simulink model "gm_sampleModel1786_sub"  (R2023a)
settings: Solver=VariableStepAuto  StartTime=0.0  StopTime=10.0  RelTol=1e-3
libraries: simulink x2
settings Model: Creator=user1  LastModifiedBy=user1
settings OptimizationCC: BlockReduction=off  ConditionallyExecuteInputs=off
settings DebuggingCC: InheritedTsInSrcMsg=none

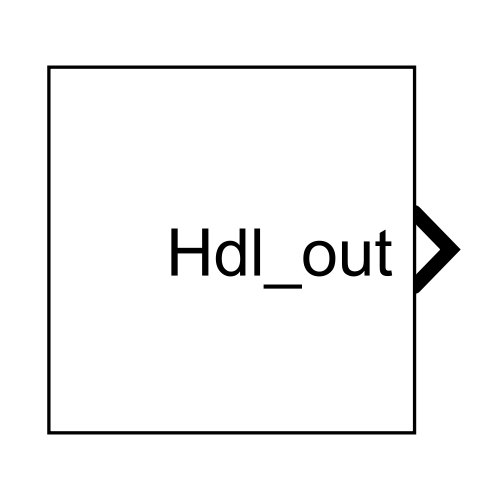
[thumbnail: Simulink's stored preview of the top-level diagram]
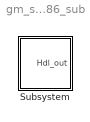
== system gm_sampleModel1786_sub ==
  Subsystem : Subsystem

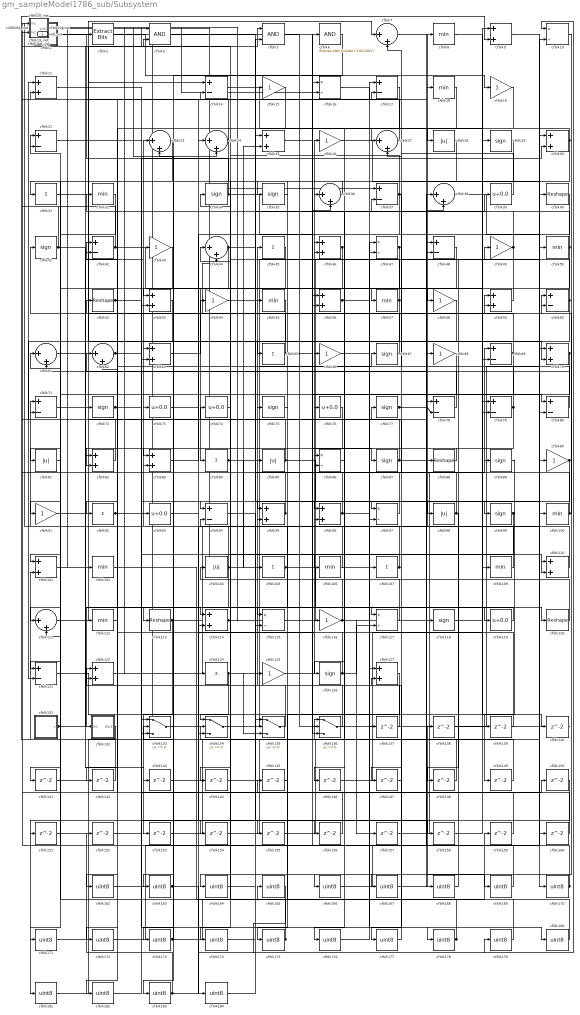
== system gm_sampleModel1786_sub/Subsystem ==
  cfblk1 : Subsystem  mask(Detect Rise Nonnegative){vinit=double(0), InputProcessing=Elements as channels (sample based), OutDataTypeStr=uint8}
      mask prompts: vinit "Simulink:masks:InitialCondition_MP"; InputProcessing "Simulink:masks:InputProcessing_MP"; OutDataTypeStr "Simulink:masks:OutputDataType_MP"
      mask help: Simulink:masks:DetectRiseNonnegative_MD
      mask init:
      | InputProcessing = 'Elements as channels (sample based)';
      | OutDataTypeStr = 'uint8';
      | vinit = double(0);
      mask TypeOptions InputProcessing: Simulink:masks:ColumnsAsChannelsFrameBased | Simulink:masks:ElementsAsChannelsSampleBased
      mask TypeOptions OutDataTypeStr: Simulink:masks:uint8 | Simulink:masks:boolean
      mask Display: fprintf('U >= 0\n&  NOT\nU/z >= 0')
  cfblk{10,16,47,86,97,115,117} (7 alike) : Product  Inputs=*/  OutDataTypeStr=uint8  RndMeth=Zero  SaturateOnIntegerOverflow=on
  cfblk{8,18,32,50,55,57,100,102,106,109,112} (11 alike) : MinMax  OutDataTypeStr=uint8
  cfblk{9,11,25,30,46,53,56,59,63,70,82..83,95..96,101,110,114,122,127} (19 alike) : Sum  OutDataTypeStr=uint8
  cfblk103_inst : Subsystem
  cfblk{28,81,85,98,104} (5 alike) : Abs  OutDataTypeStr=uint8  SaturateOnIntegerOverflow=off
  cfblk{31,45,65,84,92,105,107,124} (8 alike) : Sum  Inputs=+  OutDataTypeStr=uint8
  cfblk108_inst : Subsystem
  cfblk{7,23..24,27,36,38,44,61..62,111} (10 alike) : Sum  Inputs=|++  OutDataTypeStr=uint8
  cfblk{40,52,88,113,120} (5 alike) : Reshape
  cfblk{15,19,26,43,49,54,58,66,68,90..91,116,125} (13 alike) : Gain  OutDataTypeStr=uint8
  cfblk{29,34..35,41,67,72,75,77,87,89,99,118,126} (13 alike) : Signum
  cfblk{39,73..74,76,93,119} (6 alike) : Bias  Bias=0.0  SaturateOnIntegerOverflow=off
  cfblk{14,17,21,37,42,48,60,69,71,78..80,94,121} (14 alike) : Sum  Inputs=+-  OutDataTypeStr=uint8
  cfblk131 : Subsystem  mask(Counter Free-Running){NumBits=double(16), tsamp=double(-1)}
      mask prompts: NumBits "Simulink:masks:NumberOfBits_MP"; tsamp "Simulink:masks:SampleTime_MP"
      mask help: Simulink:masks:CounterFreeRunning_MD
  cfblk132 : Subsystem
  cfblk{133..136} (4 alike) : Switch  OutDataTypeStr=uint8  SaturateOnIntegerOverflow=off  InputSameDT=off
  cfblk{137..160} (24 alike) : Delay  SampleTime=1
  cfblk13_inst : Subsystem
  cfblk{162..184} (23 alike) : DataTypeConversion  OutDataTypeStr=uint8  SaturateOnIntegerOverflow=off  RndMeth=Floor
  cfblk2 : simulink/Logic and Bit Operations/Extract Bits  bitsToExtract=Upper half  numBits=8  bitIdxRange=[0 7]  outScalingMode=Preserve fixed-point scaling
      settings: LibrarySourceBlock=|
      | hdlsllib/Logic and Bit
      | Operations/Extract Bits
  cfblk20_inst : Subsystem
  cfblk22_inst : Subsystem
  cfblk3 : Logic  AllPortsSameDT=off  OutDataTypeStr=boolean
  cfblk4 : Constant  Value=0  OutDataTypeStr=uint8  SampleTime=1
  cfblk5 : Logic  AllPortsSameDT=off  OutDataTypeStr=boolean
  cfblk6 : simulink/Logic and Bit Operations/Bitwise Operator  logicop=AND  UseBitMask=on  BitMask=bin2dec('11011001')  BitMaskRealWorld=Stored Integer
      settings: LibrarySourceBlock=|
      | hdlsllib/Logic and Bit
      | Operations/Bitwise
      | Operator
  cfblk64_inst : Subsystem
  Hdl_out : Outport  OutDataTypeStr=uint8  SampleTime=1
  wires:
  cfblk1/1(Y) -> cfblk70/2, cfblk7/1, Hdl_out/1
  cfblk10/1 -> cfblk164/1
  cfblk100/1 -> cfblk60/1, cfblk108_inst/1(in1)
  cfblk101/1 -> cfblk5/1
  cfblk102/1 -> cfblk165/1
  cfblk103_inst/1(out1) -> cfblk72/1
  cfblk104/1 -> cfblk64_inst/2(in2), cfblk25/2, cfblk132/1(In1)
  cfblk105/1 -> cfblk67/1, cfblk120/1
  cfblk106/1 -> cfblk94/2
  cfblk107/1 -> cfblk23/1, cfblk26/1
  cfblk108_inst/1(out1) -> cfblk37/1, cfblk24/2, cfblk103_inst/2(in2)
  cfblk109/1 -> cfblk71/1
  cfblk11/1 -> cfblk53/2
  cfblk110/1 -> cfblk8/1
  cfblk111/1 -> cfblk78/1
  cfblk112/1 -> cfblk62/2
  cfblk113/1 -> cfblk153/1, cfblk117/1
  cfblk114/1 -> cfblk88/1, cfblk59/1
  cfblk115/1 -> cfblk49/1
  cfblk116/1 -> cfblk34/1, cfblk157/1
  cfblk117/1 -> cfblk76/1
  cfblk118/1 -> cfblk29/1
  cfblk119/1 -> cfblk113/1
  cfblk120/1 -> cfblk45/1
  cfblk121/1 -> cfblk149/1
  cfblk122/1 -> cfblk50/1
  cfblk124/1 -> cfblk60/2, cfblk40/1, cfblk135/3, cfblk134/1
  cfblk125/1 -> cfblk86/1
  cfblk126/1 -> cfblk52/1, cfblk117/2
  cfblk127/1 -> cfblk175/1
  cfblk13_inst/1(out1) -> cfblk16/2
  cfblk131/1(y) -> cfblk17/2, cfblk68/1
  cfblk132/1(Out1) -> cfblk9/2
  cfblk133/1 -> cfblk73/1
  cfblk134/1 -> cfblk66/1
  cfblk135/1 -> cfblk75/1
  cfblk136/1 -> cfblk42/1
  cfblk137/1 -> cfblk122/1
  cfblk138/1 -> cfblk70/1
  cfblk139/1 -> cfblk44/1
  cfblk14/1 -> cfblk109/1
  cfblk140/1 -> cfblk1/1(U)
  cfblk141/1 -> cfblk5/2
  cfblk142/1 -> cfblk101/2
  cfblk143/1 -> cfblk136/1
  cfblk144/1 -> cfblk97/2
  cfblk145/1 -> cfblk95/2
  cfblk146/1 -> cfblk9/1
  cfblk147/1 -> cfblk177/1
  cfblk148/1 -> cfblk134/2
  cfblk149/1 -> cfblk46/1
  cfblk15/1 -> cfblk183/1
  cfblk150/1 -> cfblk181/1
  cfblk151/1 -> cfblk47/2
  cfblk152/1 -> cfblk30/2
  cfblk153/1 -> cfblk136/2
  cfblk154/1 -> cfblk36/2
  cfblk155/1 -> cfblk80/2
  cfblk156/1 -> cfblk20_inst/2(in2)
  cfblk157/1 -> cfblk69/1
  cfblk158/1 -> cfblk79/1
  cfblk159/1 -> cfblk61/1
  cfblk16/1 -> cfblk137/1
  cfblk160/1 -> cfblk42/2
  cfblk162/1 -> cfblk6/1
  cfblk163/1 -> cfblk184/1, cfblk116/1
  cfblk164/1 -> cfblk89/1
  cfblk165/1 -> cfblk10/1
  cfblk166/1 -> cfblk10/2
  cfblk167/1 -> cfblk138/1
  cfblk168/1 -> cfblk48/1
  cfblk169/1 -> cfblk48/2
  cfblk17/1 -> cfblk112/1
  cfblk170/1 -> cfblk83/2, cfblk64_inst/1(in1)
  cfblk171/1 -> cfblk38/1
  cfblk172/1 -> cfblk38/2
  cfblk173/1 -> cfblk135/1, cfblk133/2, cfblk159/1
  cfblk174/1 -> cfblk55/1
  cfblk175/1 -> cfblk63/1, cfblk104/1
  cfblk176/1 -> cfblk127/1
  cfblk177/1 -> cfblk127/2
  cfblk178/1 -> cfblk71/2, cfblk145/1, cfblk125/1
  cfblk179/1 -> cfblk21/1
  cfblk18/1 -> cfblk63/2
  cfblk180/1 -> cfblk21/2
  cfblk181/1 -> cfblk115/2
  cfblk182/1 -> cfblk150/1
  cfblk183/1 -> cfblk96/2, cfblk179/1, cfblk152/1
  cfblk184/1 -> cfblk15/1
  cfblk19/1 -> cfblk126/1
  cfblk2/1 -> cfblk19/1
  cfblk20_inst/1(out1) -> cfblk135/2, cfblk107/1
  cfblk21/1 -> cfblk178/1
  cfblk22_inst/1(out1) -> cfblk102/1
  cfblk23/1 -> cfblk31/1
  cfblk24/1 -> cfblk82/2, cfblk22_inst/2(in2)
  cfblk25/1 -> cfblk28/1
  cfblk26/1 -> cfblk100/1
  cfblk27/1 -> cfblk16/1
  cfblk28/1 -> cfblk121/1
  cfblk29/1 -> cfblk65/1
  cfblk3/1 -> cfblk96/1
  cfblk30/1 -> cfblk27/1, cfblk162/1, cfblk144/1
  cfblk31/1 -> cfblk14/1
  cfblk32/1 -> cfblk151/1
  cfblk34/1 -> cfblk56/1, cfblk2/1
  cfblk35/1 -> cfblk95/1
  cfblk36/1 -> cfblk35/1
  cfblk37/1 -> cfblk3/2, cfblk134/3, cfblk97/1
  cfblk38/1 -> cfblk170/1
  cfblk39/1 -> cfblk14/2
  cfblk4/1 -> cfblk118/1
  cfblk40/1 -> cfblk166/1
  cfblk41/1 -> cfblk3/1, cfblk114/1, cfblk108_inst/2(in2)
  cfblk42/1 -> cfblk69/2, cfblk22_inst/1(in1), cfblk168/1
  cfblk43/1 -> cfblk111/2
  cfblk44/1 -> cfblk122/2, cfblk18/1
  cfblk45/1 -> cfblk53/1
  cfblk46/1 -> cfblk171/1, cfblk101/1
  cfblk47/1 -> cfblk46/2, cfblk172/1, cfblk84/1
  cfblk48/1 -> cfblk167/1
  cfblk49/1 -> cfblk182/1, cfblk32/1
  cfblk5/1 -> cfblk79/2
  cfblk50/1 -> cfblk37/2, cfblk57/1
  cfblk52/1 -> cfblk93/1, cfblk106/1
  cfblk53/1 -> cfblk141/1
  cfblk54/1 -> cfblk39/1
  cfblk55/1 -> cfblk173/1
  cfblk56/1 -> cfblk99/1, cfblk110/2
  cfblk57/1 -> cfblk136/3, cfblk13_inst/1(in1)
  cfblk58/1 -> cfblk92/1
  cfblk59/1 -> cfblk58/1
  cfblk6/1 -> cfblk163/1
  cfblk60/1 -> cfblk27/2, cfblk121/2
  cfblk61/1 -> cfblk44/2
  cfblk62/1 -> cfblk133/1, cfblk110/1
  cfblk63/1 -> cfblk54/1
  cfblk64_inst/1(out1) -> cfblk124/1
  cfblk65/1 -> cfblk87/1, cfblk25/1
  cfblk66/1 -> cfblk98/1
  cfblk67/1 -> cfblk41/1
  cfblk68/1 -> cfblk94/1
  cfblk69/1 -> cfblk81/1, cfblk91/1, cfblk47/1
  cfblk7/1 -> cfblk80/1
  cfblk70/1 -> cfblk61/2, cfblk114/2
  cfblk71/1 -> cfblk143/1
  cfblk72/1 -> cfblk59/2, cfblk30/1
  cfblk73/1 -> cfblk24/1
  cfblk74/1 -> cfblk174/1
  cfblk75/1 -> cfblk115/1
  cfblk76/1 -> cfblk83/1
  cfblk77/1 -> cfblk78/2, cfblk147/1
  cfblk78/1 -> cfblk62/1
  cfblk79/1 -> cfblk7/2, cfblk11/2, cfblk142/1
  cfblk8/1 -> cfblk140/1
  cfblk80/1 -> cfblk36/1
  cfblk81/1 -> cfblk111/1
  cfblk82/1 -> cfblk13_inst/2(in2)
  cfblk83/1 -> cfblk17/1
  cfblk84/1 -> cfblk56/2, cfblk105/1
  cfblk85/1 -> cfblk20_inst/1(in1), cfblk160/1
  cfblk86/1 -> cfblk176/1
  cfblk87/1 -> cfblk169/1, cfblk11/1
  cfblk88/1 -> cfblk82/1
  cfblk89/1 -> cfblk139/1
  cfblk9/1 -> cfblk90/1
  cfblk90/1 -> cfblk133/3, cfblk146/1
  cfblk91/1 -> cfblk43/1
  cfblk92/1 -> cfblk74/1, cfblk158/1
  cfblk93/1 -> cfblk155/1
  cfblk94/1 -> cfblk156/1
  cfblk95/1 -> cfblk85/1, cfblk23/2
  cfblk96/1 -> cfblk180/1, cfblk86/2
  cfblk97/1 -> cfblk103_inst/1(in1)
  cfblk98/1 -> cfblk77/1, cfblk148/1
  cfblk99/1 -> cfblk119/1, cfblk154/1

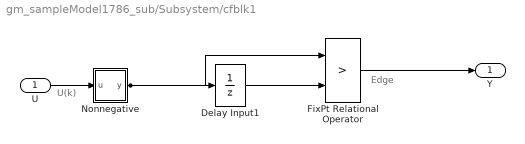
== system gm_sampleModel1786_sub/Subsystem/cfblk1 ==
  note: U(k)
  note: Edge
  U : Inport  OutDataTypeStr=uint8  SampleTime=1
  Delay Input1 : UnitDelay  Description=Store in Global RAM  DisableCoverage=on  InitialCondition=vinit  SampleTime=-1  HasFrameUpgradeWarning=on
  FixPt Relational Operator : RelationalOperator  Operator=>  OutDataTypeStr=fixdt(0, 8)  ZeroCross=off  InputSameDT=off
  Nonnegative : Subsystem  mask(Compare To Zero){relop=>=, OutDataTypeStr=boolean, ZeroCross=off}
      mask prompts: relop "Simulink:masks:Operator_MP"; OutDataTypeStr "Simulink:masks:OutputDataType_MP"; ZeroCross "Simulink:masks:EnableZerocrossingDetection_MP"
      mask help: Simulink:masks:CompareToZero_MD
      mask init:
      | OutDataTypeStr = 'boolean';
      | ZeroCross = 'off';
      | blkName = 'sampleModel1786_sub/Subsystem/cfblk1/Nonnegative';
      | relop = '>=';
      | setValue = 'boolean';
      mask TypeOptions relop: == | ~= | < | <= | >= | >
      mask TypeOptions OutDataTypeStr: Simulink:masks:uint8 | Simulink:masks:boolean
      mask Callback ZeroCross: sl('zeroCrossEnable', gcbh);
      mask Display: disp([relop,' 0'])
  Y : Outport  SampleTime=1
  wires:
  U/1 -> Nonnegative/1(u)
  Delay Input1/1 -> FixPt Relational Operator/2
  FixPt Relational Operator/1 -> Y/1
  Nonnegative/1(y) -> FixPt Relational Operator/1, Delay Input1/1

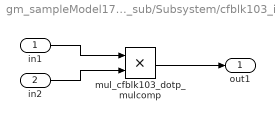
== system gm_sampleModel1786_sub/Subsystem/cfblk103_inst ==
  in1 : Inport  OutDataTypeStr=uint8  SampleTime=1
  in2 : Inport  Port=2  OutDataTypeStr=uint8  SampleTime=1
  mul_cfblk103_dotp_mulcomp : Product  Inputs=**  OutDataTypeStr=uint8  SampleTime=1
  out1 : Outport  OutDataTypeStr=uint8  SampleTime=1
  wires:
  in1/1 -> mul_cfblk103_dotp_mulcomp/1
  in2/1 -> mul_cfblk103_dotp_mulcomp/2
  mul_cfblk103_dotp_mulcomp/1 -> out1/1

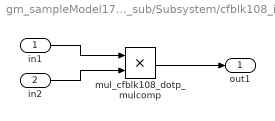
== system gm_sampleModel1786_sub/Subsystem/cfblk108_inst ==
  in1 : Inport  OutDataTypeStr=uint8  SampleTime=1
  in2 : Inport  Port=2  OutDataTypeStr=uint8  SampleTime=1
  mul_cfblk108_dotp_mulcomp : Product  Inputs=**  OutDataTypeStr=uint8  SampleTime=1
  out1 : Outport  OutDataTypeStr=uint8  SampleTime=1
  wires:
  in1/1 -> mul_cfblk108_dotp_mulcomp/1
  in2/1 -> mul_cfblk108_dotp_mulcomp/2
  mul_cfblk108_dotp_mulcomp/1 -> out1/1

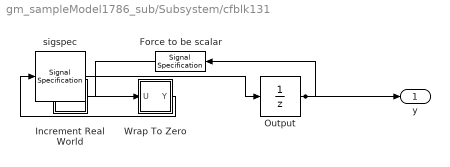
== system gm_sampleModel1786_sub/Subsystem/cfblk131 ==
  Force to be scalar : SignalSpecification  DisableCoverage=on  Dimensions=1
  Increment Real World : Subsystem  mask(Real World Value Increment){}
      mask help: Simulink:masks:RealWorldValueIncrement_MD
      mask Display: disp('V++')
  Output : UnitDelay  InitialCondition=0.0  SampleTime=tsamp  HasFrameUpgradeWarning=on
  Wrap To Zero : Subsystem  mask(Wrap To Zero){Threshold=double(65535)}
      mask prompts: Threshold "Simulink:masks:Threshold_MP"
      mask help: Simulink:masks:WrapToZero_MD
  sigspec : SignalSpecification  OutDataTypeStr=uint16  Dimensions=1
  y : Outport  SampleTime=1
  wires:
  Force to be scalar/1 -> Increment Real World/1(u)
  Increment Real World/1(y) -> Wrap To Zero/1(U)
  Output/1 -> Force to be scalar/1, y/1
  Wrap To Zero/1(Y) -> sigspec/1
  sigspec/1 -> Output/1

== system gm_sampleModel1786_sub/Subsystem/cfblk132 ==
  In1 : Inport  OutDataTypeStr=uint8  PortDimensions=1  SampleTime=1
  Out1 : Outport  SampleTime=1
  wires:
  In1/1 -> Out1/1

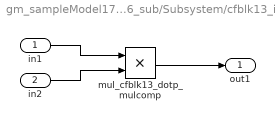
== system gm_sampleModel1786_sub/Subsystem/cfblk13_inst ==
  in1 : Inport  OutDataTypeStr=uint8  SampleTime=1
  in2 : Inport  Port=2  OutDataTypeStr=uint8  SampleTime=1
  mul_cfblk13_dotp_mulcomp : Product  Inputs=**  OutDataTypeStr=uint8  SampleTime=1
  out1 : Outport  OutDataTypeStr=uint8  SampleTime=1
  wires:
  in1/1 -> mul_cfblk13_dotp_mulcomp/1
  in2/1 -> mul_cfblk13_dotp_mulcomp/2
  mul_cfblk13_dotp_mulcomp/1 -> out1/1

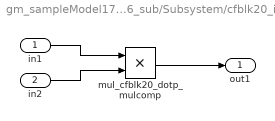
== system gm_sampleModel1786_sub/Subsystem/cfblk20_inst ==
  in1 : Inport  OutDataTypeStr=uint8  SampleTime=1
  in2 : Inport  Port=2  OutDataTypeStr=uint8  SampleTime=1
  mul_cfblk20_dotp_mulcomp : Product  Inputs=**  OutDataTypeStr=uint8  SampleTime=1
  out1 : Outport  OutDataTypeStr=uint8  SampleTime=1
  wires:
  in1/1 -> mul_cfblk20_dotp_mulcomp/1
  in2/1 -> mul_cfblk20_dotp_mulcomp/2
  mul_cfblk20_dotp_mulcomp/1 -> out1/1

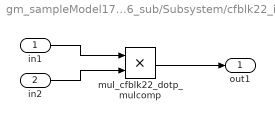
== system gm_sampleModel1786_sub/Subsystem/cfblk22_inst ==
  in1 : Inport  OutDataTypeStr=uint8  SampleTime=1
  in2 : Inport  Port=2  OutDataTypeStr=uint8  SampleTime=1
  mul_cfblk22_dotp_mulcomp : Product  Inputs=**  OutDataTypeStr=uint8  SampleTime=1
  out1 : Outport  OutDataTypeStr=uint8  SampleTime=1
  wires:
  in1/1 -> mul_cfblk22_dotp_mulcomp/1
  in2/1 -> mul_cfblk22_dotp_mulcomp/2
  mul_cfblk22_dotp_mulcomp/1 -> out1/1

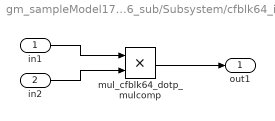
== system gm_sampleModel1786_sub/Subsystem/cfblk64_inst ==
  in1 : Inport  OutDataTypeStr=uint8  SampleTime=1
  in2 : Inport  Port=2  OutDataTypeStr=uint8  SampleTime=1
  mul_cfblk64_dotp_mulcomp : Product  Inputs=**  OutDataTypeStr=uint8  SampleTime=1
  out1 : Outport  OutDataTypeStr=uint8  SampleTime=1
  wires:
  in1/1 -> mul_cfblk64_dotp_mulcomp/1
  in2/1 -> mul_cfblk64_dotp_mulcomp/2
  mul_cfblk64_dotp_mulcomp/1 -> out1/1

== system gm_sampleModel1786_sub/Subsystem/cfblk1/Nonnegative ==
  u : Inport  OutDataTypeStr=uint8  SampleTime=1
  Compare : RelationalOperator  OutDataTypeStr=boolean  ZeroCross=off
  Constant : Constant  DisableCoverage=on  Value=0  OutDataTypeStr=Inherit: Inherit via back propagation  SampleTime=-1  PreserveConstantTs=on
  y : Outport  SampleTime=1
  wires:
  u/1 -> Compare/1
  Compare/1 -> y/1
  Constant/1 -> Compare/2

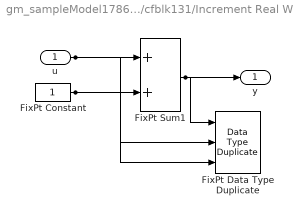
== system gm_sampleModel1786_sub/Subsystem/cfblk131/Increment Real World ==
  u : Inport  OutDataTypeStr=uint16  SampleTime=1
  FixPt Constant : Constant  DisableCoverage=on  OutDataTypeStr=Inherit: Inherit via back propagation  SampleTime=-1
  FixPt Data Type Duplicate : DataTypeDuplicate  DisableCoverage=on  NumInputPorts=3
  FixPt Sum1 : Sum  InputSameDT=on  OutDataTypeStr=Inherit: Inherit via back propagation  LockScale=on
  y : Outport  SampleTime=1
  wires:
  u/1 -> FixPt Sum1/1, FixPt Data Type Duplicate/2
  FixPt Constant/1 -> FixPt Sum1/2, FixPt Data Type Duplicate/3
  FixPt Sum1/1 -> FixPt Data Type Duplicate/1, y/1

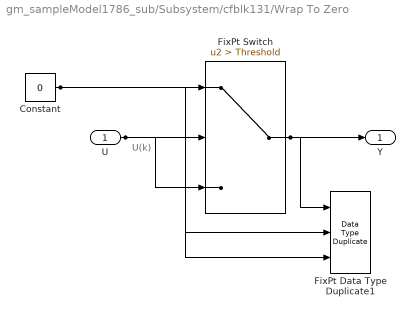
== system gm_sampleModel1786_sub/Subsystem/cfblk131/Wrap To Zero ==
  note: U(k)
  U : Inport  OutDataTypeStr=uint16  SampleTime=1
  Constant : Constant  DisableCoverage=on  Value=0  OutDataTypeStr=Inherit: Inherit via back propagation  SampleTime=-1
  FixPt Data Type Duplicate1 : DataTypeDuplicate  DisableCoverage=on  NumInputPorts=3
  FixPt Switch : Switch  Criteria=u2 > Threshold  Threshold=Threshold  OutDataTypeStr=Inherit: Inherit via back propagation  ZeroCross=off  SaturateOnIntegerOverflow=off  InputSameDT=off
  Y : Outport  SampleTime=1
  wires:
  U/1 -> FixPt Switch/3, FixPt Switch/2, FixPt Data Type Duplicate1/2
  Constant/1 -> FixPt Switch/1, FixPt Data Type Duplicate1/3
  FixPt Switch/1 -> FixPt Data Type Duplicate1/1, Y/1
